simulink model "coulumb_counting"  (R2022a)
settings: Solver=FixedStepAuto  StartTime=0.0  StopTime=3600  FixedStep=0.01  RelTol=1e-3
libraries: simulink_extras x1
settings Model: Creator=10661025  LastModifiedBy=10661025

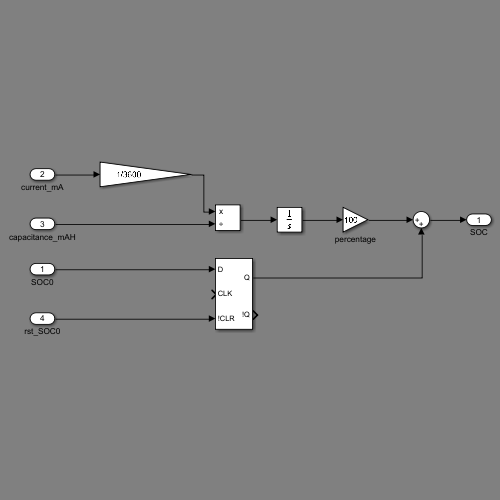
[thumbnail: Simulink's stored preview of the top-level diagram]
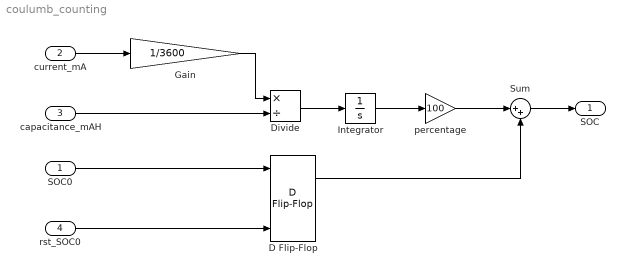
== system coulumb_counting ==
  SOC0 : Inport
  current_mA : Inport  Port=2
  capacitance_mAH : Inport  Port=3
  rst_SOC0 : Inport  Port=4
  D Flip-Flop : simulink_extras/Flip Flops/D Flip-Flop
  Divide : Product  Inputs=*/
  Gain : Gain  Gain=1/3600
  Integrator : Integrator
  Sum : Sum  Inputs=|++
  percentage : Gain  Gain=100
  SOC : Outport
  wires:
  current_mA/1 -> Gain/1
  Integrator/1 -> percentage/1
  Gain/1 -> Divide/1
  Sum/1 -> SOC/1
  SOC0/1 -> D Flip-Flop/1
  percentage/1 -> Sum/1
  capacitance_mAH/1 -> Divide/2
  Divide/1 -> Integrator/1
  rst_SOC0/1 -> D Flip-Flop/3
  D Flip-Flop/1 -> Sum/2
